simulink model "fado_external_observer_wrapper"  (R2026a)
settings: Solver=FixedStepDiscrete  FixedStep=5e-5
settings Model: Creator=hzldx  LastModifiedBy=hzldx
settings HardwareCC: ProdLargestAtomicInteger=Long  ProdLargestAtomicFloat=Double  ProdHWDeviceType=ARM Compatible->ARM Cortex-M
settings RTWCC: SystemTargetFile=ert.tlc  GenCodeOnly=on  GenerateMakefile=off  Description=Embedded Coder

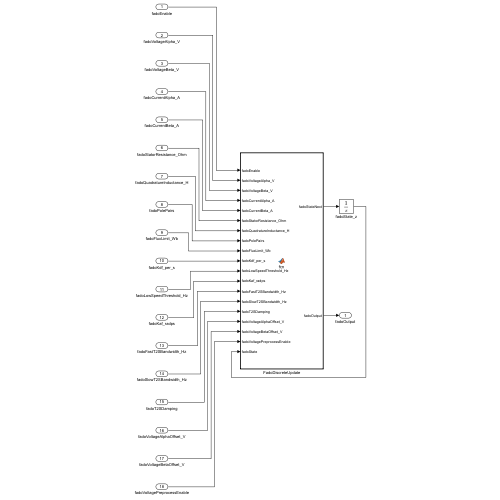
[thumbnail: Simulink's stored preview of the top-level diagram]
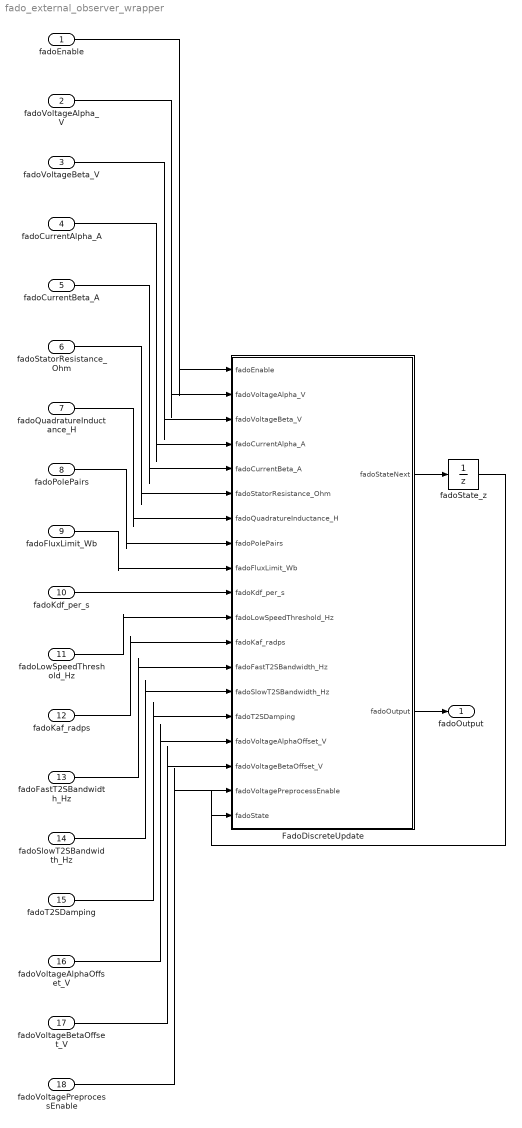
== system fado_external_observer_wrapper ==
  fadoEnable : Inport  OutDataTypeStr=boolean
  fadoVoltageAlpha_V : Inport  Port=2  OutDataTypeStr=single
  fadoVoltageBeta_V : Inport  Port=3  OutDataTypeStr=single
  fadoCurrentAlpha_A : Inport  Port=4  OutDataTypeStr=single
  fadoCurrentBeta_A : Inport  Port=5  OutDataTypeStr=single
  fadoStatorResistance_Ohm : Inport  Port=6  OutDataTypeStr=single
  fadoQuadratureInductance_H : Inport  Port=7  OutDataTypeStr=single
  fadoPolePairs : Inport  Port=8  OutDataTypeStr=uint8
  fadoFluxLimit_Wb : Inport  Port=9  OutDataTypeStr=single
  fadoKdf_per_s : Inport  Port=10  OutDataTypeStr=single
  fadoLowSpeedThreshold_Hz : Inport  Port=11  OutDataTypeStr=single
  fadoKaf_radps : Inport  Port=12  OutDataTypeStr=single
  fadoFastT2SBandwidth_Hz : Inport  Port=13  OutDataTypeStr=single
  fadoSlowT2SBandwidth_Hz : Inport  Port=14  OutDataTypeStr=single
  fadoT2SDamping : Inport  Port=15  OutDataTypeStr=single
  fadoVoltageAlphaOffset_V : Inport  Port=16  OutDataTypeStr=single
  fadoVoltageBetaOffset_V : Inport  Port=17  OutDataTypeStr=single
  fadoVoltagePreprocessEnable : Inport  Port=18  OutDataTypeStr=boolean
  FadoDiscreteUpdate : MATLAB Function  TreatAsAtomicUnit=on
  fadoState_z : UnitDelay  InitialCondition=zeros(10,1)  SampleTime=5e-5  StateName=fadoState_z
  fadoOutput : Outport
  wires:
  FadoDiscreteUpdate/2(fadoOutput) -> fadoOutput/1
  FadoDiscreteUpdate/1(fadoStateNext) -> fadoState_z/1
  fadoState_z/1 -> FadoDiscreteUpdate/19(fadoState)
  fadoVoltagePreprocessEnable/1 -> FadoDiscreteUpdate/18(fadoVoltagePreprocessEnable)
  fadoVoltageBetaOffset_V/1 -> FadoDiscreteUpdate/17(fadoVoltageBetaOffset_V)
  fadoVoltageAlphaOffset_V/1 -> FadoDiscreteUpdate/16(fadoVoltageAlphaOffset_V)
  fadoT2SDamping/1 -> FadoDiscreteUpdate/15(fadoT2SDamping)
  fadoSlowT2SBandwidth_Hz/1 -> FadoDiscreteUpdate/14(fadoSlowT2SBandwidth_Hz)
  fadoFastT2SBandwidth_Hz/1 -> FadoDiscreteUpdate/13(fadoFastT2SBandwidth_Hz)
  fadoKaf_radps/1 -> FadoDiscreteUpdate/12(fadoKaf_radps)
  fadoLowSpeedThreshold_Hz/1 -> FadoDiscreteUpdate/11(fadoLowSpeedThreshold_Hz)
  fadoKdf_per_s/1 -> FadoDiscreteUpdate/10(fadoKdf_per_s)
  fadoFluxLimit_Wb/1 -> FadoDiscreteUpdate/9(fadoFluxLimit_Wb)
  fadoPolePairs/1 -> FadoDiscreteUpdate/8(fadoPolePairs)
  fadoQuadratureInductance_H/1 -> FadoDiscreteUpdate/7(fadoQuadratureInductance_H)
  fadoStatorResistance_Ohm/1 -> FadoDiscreteUpdate/6(fadoStatorResistance_Ohm)
  fadoCurrentBeta_A/1 -> FadoDiscreteUpdate/5(fadoCurrentBeta_A)
  fadoCurrentAlpha_A/1 -> FadoDiscreteUpdate/4(fadoCurrentAlpha_A)
  fadoVoltageBeta_V/1 -> FadoDiscreteUpdate/3(fadoVoltageBeta_V)
  fadoVoltageAlpha_V/1 -> FadoDiscreteUpdate/2(fadoVoltageAlpha_V)
  fadoEnable/1 -> FadoDiscreteUpdate/1(fadoEnable)

== matlab function fado_external_observer_wrapper/FadoDiscreteUpdate ==
  data: fadoEnable input boolean size=1; fadoStateNext output single size=[10 1]; fadoVoltageAlpha_V input single size=1; fadoVoltageBeta_V input single size=1; fadoCurrentAlpha_A input single size=1; fadoCurrentBeta_A input single size=1; fadoStatorResistance_Ohm input single size=1; fadoQuadratureInductance_H input single size=1; fadoPolePairs input uint8 size=1; fadoFluxLimit_Wb input single size=1; fadoKdf_per_s input single size=1; fadoLowSpeedThreshold_Hz input single size=1; fadoKaf_radps input single size=1; fadoFastT2SBandwidth_Hz input single size=1; fadoSlowT2SBandwidth_Hz input single size=1; fadoT2SDamping input single size=1; fadoVoltageAlphaOffset_V input single size=1; fadoVoltageBetaOffset_V input single size=1; fadoVoltagePreprocessEnable input boolean size=1; fadoState input single size=[10 1]; fadoOutput output single size=[18 1]
function [fadoStateNext, fadoOutput] = fcn(fadoEnable, fadoVoltageAlpha_V, fadoVoltageBeta_V, fadoCurrentAlpha_A, fadoCurrentBeta_A, fadoStatorResistance_Ohm, fadoQuadratureInductance_H, fadoPolePairs, fadoFluxLimit_Wb, fadoKdf_per_s, fadoLowSpeedThreshold_Hz, fadoKaf_radps, fadoFastT2SBandwidth_Hz, fadoSlowT2SBandwidth_Hz, fadoT2SDamping, fadoVoltageAlphaOffset_V, fadoVoltageBetaOffset_V, fadoVoltagePreprocessEnable, fadoState)
%#codegen
[fadoStateNext, fadoOutput] = fado_external_observer_discrete_update(fadoEnable, fadoVoltageAlpha_V, fadoVoltageBeta_V, fadoCurrentAlpha_A, fadoCurrentBeta_A, fadoStatorResistance_Ohm, fadoQuadratureInductance_H, fadoPolePairs, fadoFluxLimit_Wb, fadoKdf_per_s, fadoLowSpeedThreshold_Hz, fadoKaf_radps, fadoFastT2SBandwidth_Hz, fadoSlowT2SBandwidth_Hz, fadoT2SDamping, fadoVoltageAlphaOffset_V, fadoVoltageBetaOffset_V, fadoVoltagePreprocessEnable, fadoState);
end
